simulink model "simulink_wahadlo"  (R2022b)
settings: Solver=VariableStepAuto  StartTime=0.0  StopTime=100  RelTol=1e-3
values from neighbouring files (symbols this model uses):
  A = [0, g * (M + m) / (M * L), b / (M * L), 0 ... (first row only)    [wahadlo.m]
  B = [-1/(M * L) ... (first row only)    [wahadlo.m]
  C = diag([1 1 1 1])    [wahadlo.m]
  K = lqr(A,B,Q,R)    [wahadlo.m]
  x = [0;0;0;1]")    [wahadlo.m]
settings Model: Creator=wojna  LastModifiedBy=adasiak

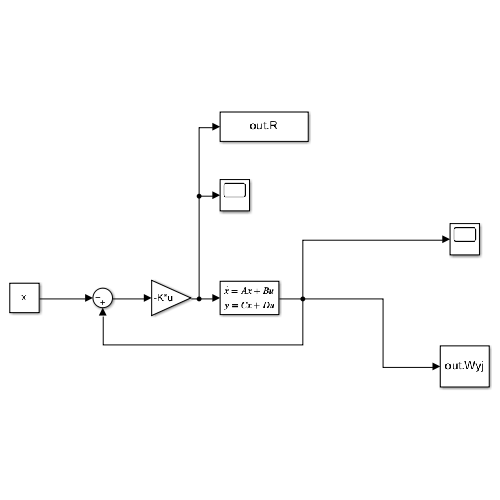
[thumbnail: Simulink's stored preview of the top-level diagram]
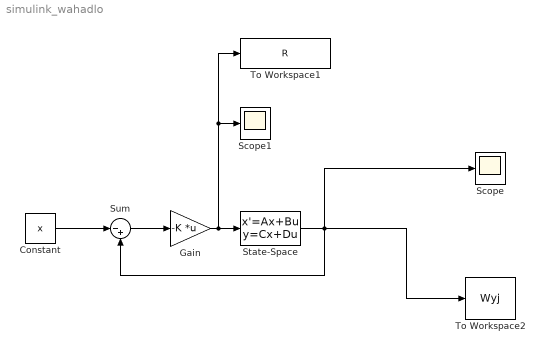
== system simulink_wahadlo ==
  Constant : Constant  Value=x  SampleTime=1
  Gain : Gain  Gain=-K  Multiplication=Matrix(K*u)
  Scope : Scope
  Scope1 : Scope
  State-Space : StateSpace  A=A  B=B  C=C  D=[0;0;0;0]  InitialCondition=0
  Sum : Sum  Inputs=|-+
  To Workspace1 : ToWorkspace  VariableName=R  SampleTime=-1
  To Workspace2 : ToWorkspace  VariableName=Wyj  SampleTime=-1
  wires:
  Gain/1 -> To Workspace1/1, Scope1/1, State-Space/1
  State-Space/1 -> Sum/2, To Workspace2/1, Scope/1
  Sum/1 -> Gain/1
  Constant/1 -> Sum/1
